simulink model "w1p4"  (R2020b)
settings: Solver=VariableStepAuto  StartTime=0.0  StopTime=10.0  RelTol=1e-3
settings Model: Creator=family  LastModifiedBy=family

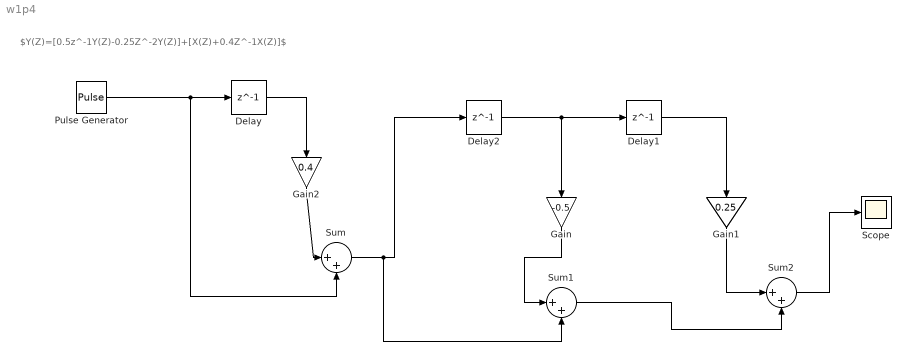
== system w1p4 ==
  note: $Y(Z)=[0.5z^-1Y(Z)-0.25Z^-2Y(Z)]+[X(Z)+0.4Z^-1X(Z)]$
  Delay : Delay  DelayLength=1
  Delay1 : Delay  DelayLength=1
  Delay2 : Delay  DelayLength=1
  Gain : Gain  Gain=-0.5
  Gain1 : Gain  Gain=0.25
  Gain2 : Gain  Gain=0.4
  Pulse Generator : DiscretePulseGenerator  PulseType=Time based  Period=10  PulseWidth=5
  Scope : Scope
  Sum : Sum  Inputs=|++
  Sum1 : Sum  Inputs=|++
  Sum2 : Sum  Inputs=|++
  wires:
  Pulse Generator/1 -> Sum/2, Delay/1
  Delay/1 -> Gain2/1
  Gain2/1 -> Sum/1
  Sum/1 -> Sum1/2, Delay2/1
  Delay2/1 -> Gain/1, Delay1/1
  Delay1/1 -> Gain1/1
  Gain1/1 -> Sum2/1
  Gain/1 -> Sum1/1
  Sum1/1 -> Sum2/2
  Sum2/1 -> Scope/1
